simulink model "model_estimation"  (R2020b)
settings: Solver=VariableStepAuto  StartTime=0.0  StopTime=10.0  RelTol=1e-3
values from neighbouring files (symbols this model uses):
  Cx = 1.15    [main.m]
  p_0 = 1    [main.m]
  p_1 = 1    [main.m]
  p_2 = 1    [main.m]
  rho = 1.2    [main.m]
settings Model: OrderedModelArguments=off  Creator=artem  LastModifiedBy=artem

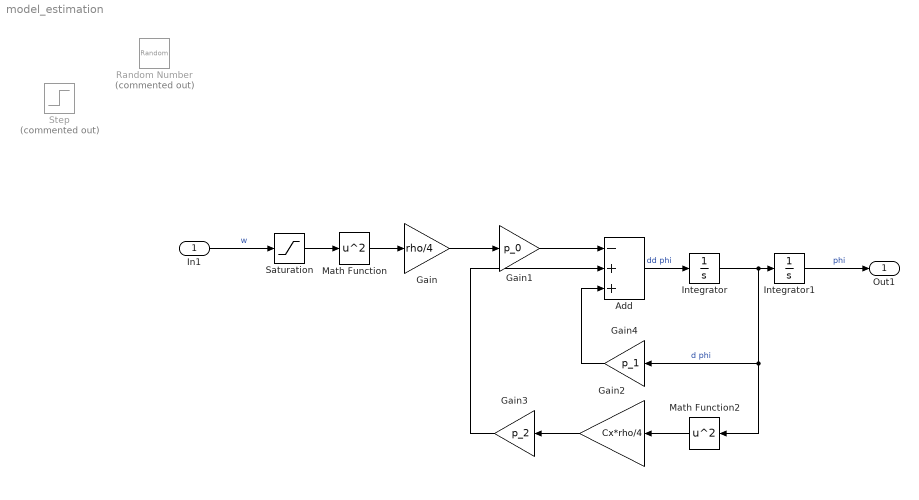
== system model_estimation ==
  In1 : Inport
  Add : Sum  Inputs=-++
  Gain : Gain  Gain=rho/4
  Gain1 : Gain  Gain=p_0
  Gain2 : Gain  Gain=Cx*rho/4
  Gain3 : Gain  Gain=p_2
  Gain4 : Gain  Gain=p_1
  Integrator : Integrator
  Integrator1 : Integrator
  Math Function : Math  Operator=square  SaturateOnIntegerOverflow=on
  Math Function2 : Math  Operator=square  SaturateOnIntegerOverflow=on
  Random Number : RandomNumber  Commented=on  SampleTime=0.1
  Saturation : Saturate  UpperLimit=125  LowerLimit=-125
  Step : Step  Commented=on  SampleTime=0
  Out1 : Outport
  wires:
  Math Function/1 -> Gain/1
  Gain1/1 -> Add/1
  Gain/1 -> Gain1/1
  Gain3/1 -> Add/2
  Gain4/1 -> Add/3
  Saturation/1 -> Math Function/1
  Add/1 -> Integrator/1  "dd phi"
  Gain2/1 -> Gain3/1
  In1/1 -> Saturation/1  "w"
  Integrator/1 -> Math Function2/1, Gain4/1, Integrator1/1  "d phi"
  Integrator1/1 -> Out1/1  "phi"
  Math Function2/1 -> Gain2/1
